simulink model "MCU_CmdTransV3"  (R2022b)
settings: Solver=FixedStepDiscrete  StartTime=0.0  StopTime=10.0  FixedStep=0.001  RelTol=1e-3
undefined symbols (not defined in the file or in its folder): ANALOG, cAgeingMode, cCurrentLoopMode, cNoneMode, cParaRecogMode, cSingleBoardMode, cSpeedLoopMode, cTorqueLoopMode, cVvvfOpenMode, FAULT, ParamCfg_CommandSource_u16, ParamCfg_MaxSpeed_u16, ParamCfg_MaxTorque_u16, ParamCfg_Spdouttype_u16, ParamCfg_Vc1Enable_u16, POWER_ON, STANDBY, TESTBED, VEHICLE
libraries: simulink x8
(part 1 of 2)
settings Model: DataDictionary=MCU_CmdTransV2_objects.sldd  Creator=ZYH  LastModifiedBy=ZYH
settings OptimizationCC: DefaultParameterBehavior=Inlined  EnhancedBackFolding=on  PassReuseOutputArgsAs=Individual arguments  OptimizeBlockOrder=speed  DifferentSizesBufferReuse=on  OptimizationCustomize=off  EfficientTunableParamExpr=on
settings DebuggingCC: ParameterTunabilityLossMsg=error
settings SFSimCC: MATLABDynamicMemAlloc=off
settings RTWCC: Description=Embedded Coder  SystemTargetFile=ert.tlc  GenCodeOnly=on  TemplateMakefile=ert_default_tmf
settings CodeAppCC: ForceParamTrailComments=on  IgnoreCustomStorageClasses=off  OperatorAnnotations=on  SimulinkDataObjDesc=on  SFDataObjDesc=on  InsertBlockDesc=on
settings ERTTargetCC: TargetLangStandard=C99 (ISO)  GenerateSampleERTMain=on  InlinedParameterPlacement=NonHierarchical  ERTCustomFileTemplate=example_file_process.tlc

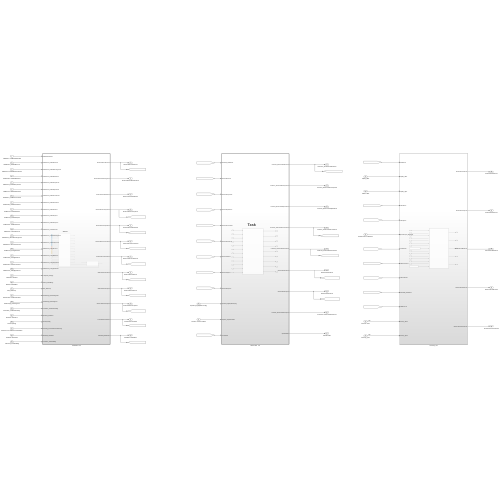
[thumbnail: Simulink's stored preview of the top-level diagram]
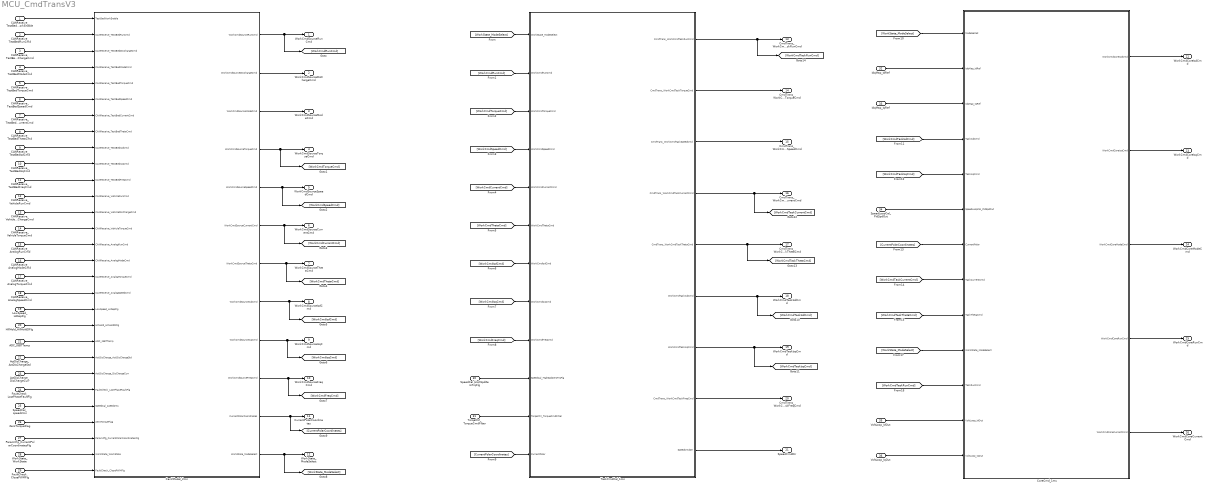
== system MCU_CmdTransV3 ==
  CANReceive_TestBedWorkEnable : Inport
  CANReceive_TestBedRunCmd : Inport  Port=2
  CANReceive_TestBedDisChargeCmd : Inport  Port=3
  CANReceive_TestBedModeCmd : Inport  Port=4
  CANReceive_TestBedTorqueCmd : Inport  Port=5
  CANReceive_TestBedSpeedCmd : Inport  Port=6
  CANReceive_TestBedCurrentCmd : Inport  Port=7
  CANReceive_TestBedThetaCmd : Inport  Port=8
  CANReceive_TestBedIsdCmd : Inport  Port=9
  CANReceive_TestBedIsqCmd : Inport  Port=10
  CANReceive_TestBedFreqCmd : Inport  Port=11
  CANReceive_VehicleRunCmd : Inport  Port=12
  CANReceive_VehicleDisChargeCmd : Inport  Port=13
  CANReceive_VehicleTorqueCmd : Inport  Port=14
  CANReceive_AnalogRunCmd : Inport  Port=15
  CANReceive_AnalogModeCmd : Inport  Port=16
  CANReceive_AnalogTorqueCmd : Inport  Port=17
  CANReceive_AnalogSpeedCmd : Inport  Port=18
  LowSpeed_LsDepFlg : Inport  Port=19
  HillHold_HillHoldDFlg : Inport  Port=20
  ADC_IGBTTemp : Inport  Port=21
  ActDisCharge_ActDisChargeStd : Inport  Port=22
  ActDisCharge_DisChargeCurr : Inport  Port=23
  FaultCheck_LostPhaseFaultFlg : Inport  Port=24
  SpeedCal_speed2ms : Inport  Port=25
  ZeroTorqueFlag : Inport  Port=26
  ParamCfg_CurrentPolarCoordinatesFlg : Inport  Port=27
  WorkState_WorkState : Inport  Port=28
  FaultCheck_ClosePWMFlg : Inport  Port=29
  SpeedCal_HighSpdZeroTrqFlg : Inport  Port=30
  TorqeCtrl_TorqueCmdFilter : Inport  Port=31
  IdqMap_IdRef : Inport  Port=32
  IdqMap_IqRef : Inport  Port=33
  SpeedLoopCal_PidSpdOut : Inport  Port=34
  VoltLoop_IdOut : Inport  Port=35  OutDataTypeStr=single
  VoltLoop_IqOut : Inport  Port=36  OutDataTypeStr=single
  Can2Model_2ms : Subsystem  TreatAsAtomicUnit=on
  CoreCmd_1ms : Subsystem
  TaskCmdCal_1ms : Subsystem  TreatAsAtomicUnit=on
  WorkCmdSourceRunCmd : Outport
  WorkCmdSourceDisChargeCmd : Outport  Port=2
  WorkCmdSourceModeCmd : Outport  Port=3
  WorkCmdSourceTorqueCmd : Outport  Port=4
  WorkCmdSourceSpeedCmd : Outport  Port=5
  WorkCmdSourceCurrentCmd : Outport  Port=6
  WorkCmdSourceThetaCmd : Outport  Port=7
  WorkCmdSourceIsdCmd : Outport  Port=8
  WorkCmdSourceIsqCmd : Outport  Port=9
  WorkCmdSourceFreqCmd : Outport  Port=10
  CurrentPolarCoordinates : Outport  Port=11
  WorkState_ModeSelect : Outport  Port=12
  CmdTrans_WorkCmdTaskRunCmd : Outport  Port=13
  CmdTrans_WorkCmdTaskTorqueCmd : Outport  Port=14
  CmdTrans_WorkCmdTaskSpeedCmd : Outport  Port=15
  CmdTrans_WorkCmdTaskCurrentCmd : Outport  Port=16
  CmdTrans_WorkCmdTaskThetaCmd : Outport  Port=17
  WorkCmdTaskIsdCmd : Outport  Port=18
  WorkCmdTaskIsqCmd : Outport  Port=19
  CmdTrans_WorkCmdTaskFreqCmd : Outport  Port=20
  SpeedCmdDir : Outport  Port=21
  WorkCmdCoreIsdCmd : Outport  Port=22
  WorkCmdCoreIsqCmd : Outport  Port=23
  WorkCmdCoreModeCmd : Outport  Port=24
  WorkCmdCoreRunCmd : Outport  Port=25
  WorkCmdCoreCurrentCmd : Outport  Port=26
  wires:
  CANReceive_TestBedModeCmd/1 -> Can2Model_2ms/4(CANReceive_TestBedModeCmd)
  CANReceive_TestBedTorqueCmd/1 -> Can2Model_2ms/5(CANReceive_TestBedTorqueCmd)
  CANReceive_TestBedDisChargeCmd/1 -> Can2Model_2ms/3(CANReceive_TestBedDisChargeCmd)
  CANReceive_TestBedWorkEnable/1 -> Can2Model_2ms/1(TestBedWorkEnable)
  CANReceive_TestBedRunCmd/1 -> Can2Model_2ms/2(CANReceive_TestBedRunCmd)
  CANReceive_TestBedIsdCmd/1 -> Can2Model_2ms/9(CANReceive_TestBedIsdCmd)
  CANReceive_TestBedIsqCmd/1 -> Can2Model_2ms/10(CANReceive_TestBedIsqCmd)
  CANReceive_TestBedThetaCmd/1 -> Can2Model_2ms/8(CANReceive_TestBedThetaCmd)
  CANReceive_TestBedFreqCmd/1 -> Can2Model_2ms/11(CANReceive_TestBedFreqCmd)
  CANReceive_VehicleRunCmd/1 -> Can2Model_2ms/12(CANReceive_VehicleRunCmd)
  CANReceive_VehicleDisChargeCmd/1 -> Can2Model_2ms/13(CANReceive_VehicleDisChargeCmd)
  CANReceive_TestBedCurrentCmd/1 -> Can2Model_2ms/7(CANReceive_TestBedCurrentCmd)
  CANReceive_TestBedSpeedCmd/1 -> Can2Model_2ms/6(CANReceive_TestBedSpeedCmd)
  CANReceive_AnalogTorqueCmd/1 -> Can2Model_2ms/17(CANReceive_AnalogTorqueCmd)
  CANReceive_AnalogSpeedCmd/1 -> Can2Model_2ms/18(CANReceive_AnalogSpeedCmd)
  CANReceive_AnalogModeCmd/1 -> Can2Model_2ms/16(CANReceive_AnalogModeCmd)
  LowSpeed_LsDepFlg/1 -> Can2Model_2ms/19(LowSpeed_LsDepFlg)
  CANReceive_AnalogRunCmd/1 -> Can2Model_2ms/15(CANReceive_AnalogRunCmd)
  CANReceive_VehicleTorqueCmd/1 -> Can2Model_2ms/14(CANReceive_VehicleTorqueCmd)
  ActDisCharge_ActDisChargeStd/1 -> Can2Model_2ms/22(ActDisCharge_ActDisChargeStd)
  ActDisCharge_DisChargeCurr/1 -> Can2Model_2ms/23(ActDisCharge_DisChargeCurr)
  FaultCheck_LostPhaseFaultFlg/1 -> Can2Model_2ms/24(FaultCheck_LostPhaseFaultFlg)
  Can2Model_2ms/1(WorkCmdSourceRunCmd) -> [WorkCmdRunCmd], WorkCmdSourceRunCmd/1
  Can2Model_2ms/2(WorkCmdSourceDisChargeCmd) -> WorkCmdSourceDisChargeCmd/1
  Can2Model_2ms/3(WorkCmdSourceModeCmd) -> WorkCmdSourceModeCmd/1
  Can2Model_2ms/4(WorkCmdSourceTorqueCmd) -> [WorkCmdTorqueCmd], WorkCmdSourceTorqueCmd/1
  Can2Model_2ms/5(WorkCmdSourceSpeedCmd) -> WorkCmdSourceSpeedCmd/1, [WorkCmdSpeedCmd]
  Can2Model_2ms/6(WorkCmdSourceCurrentCmd) -> WorkCmdSourceCurrentCmd/1, [WorkCmdCurrentCmd]
  Can2Model_2ms/7(WorkCmdSourceThetaCmd) -> WorkCmdSourceThetaCmd/1, [WorkCmdThetaCmd]
  Can2Model_2ms/8(WorkCmdSourceIsdCmd) -> WorkCmdSourceIsdCmd/1, [WorkCmdIsdCmd]
  Can2Model_2ms/9(WorkCmdSourceIsqCmd) -> [WorkCmdIsqCmd], WorkCmdSourceIsqCmd/1
  Can2Model_2ms/11(CurrentPolarCoordinates) -> [CurrentPolarCoordinates], CurrentPolarCoordinates/1
  Can2Model_2ms/10(WorkCmdSourceFreqCmd) -> [WorkCmdFreqCmd], WorkCmdSourceFreqCmd/1
  ParamCfg_CurrentPolarCoordinatesFlg/1 -> Can2Model_2ms/27(ParamCfg_CurrentPolarCoordinatesFlg)
  ZeroTorqueFlag/1 -> Can2Model_2ms/26(ZeroTorqueFlag)
  SpeedCal_speed2ms/1 -> Can2Model_2ms/25(SpeedCal_speed2ms)
  WorkState_WorkState/1 -> Can2Model_2ms/28(WorkState_WorkState)
  FaultCheck_ClosePWMFlg/1 -> Can2Model_2ms/29(FaultCheck_ClosePWMFlg)
  Can2Model_2ms/12(WorkState_ModeSelect) -> [WorkState_ModeSelect], WorkState_ModeSelect/1
  [WorkState_ModeSelect] -> TaskCmdCal_1ms/1(WorkState_ModeSelect)
  [WorkCmdRunCmd] -> TaskCmdCal_1ms/2(WorkCmdRunCmd)
  [WorkCmdTorqueCmd] -> TaskCmdCal_1ms/3(WorkCmdTorqueCmd)
  [WorkCmdSpeedCmd] -> TaskCmdCal_1ms/4(WorkCmdSpeedCmd)
  [WorkCmdCurrentCmd] -> TaskCmdCal_1ms/5(WorkCmdCurrentCmd)
  [WorkCmdThetaCmd] -> TaskCmdCal_1ms/6(WorkCmdThetaCmd)
  [WorkCmdIsdCmd] -> TaskCmdCal_1ms/7(WorkCmdIsdCmd)
  [WorkCmdIsqCmd] -> TaskCmdCal_1ms/8(WorkCmdIsqCmd)
  [WorkCmdFreqCmd] -> TaskCmdCal_1ms/9(WorkCmdFreqCmd)
  SpeedCal_HighSpdZeroTrqFlg/1 -> TaskCmdCal_1ms/10(SpeedCal_HighSpdZeroTrqFlg)
  TorqeCtrl_TorqueCmdFilter/1 -> TaskCmdCal_1ms/11(TorqeCtrl_TorqueCmdFilter)
  [CurrentPolarCoordinates] -> TaskCmdCal_1ms/12(CurrentPolar)
  HillHold_HillHoldDFlg/1 -> Can2Model_2ms/20(HillHold_HillHoldDFlg)
  ADC_IGBTTemp/1 -> Can2Model_2ms/21(ADC_IGBTTemp)
  TaskCmdCal_1ms/9(SpeedCmdDir) -> SpeedCmdDir/1
  TaskCmdCal_1ms/3(CmdTrans_WorkCmdTaskSpeedCmd) -> CmdTrans_WorkCmdTaskSpeedCmd/1
  TaskCmdCal_1ms/8(CmdTrans_WorkCmdTaskFreqCmd) -> CmdTrans_WorkCmdTaskFreqCmd/1
  TaskCmdCal_1ms/6(WorkCmdTaskIsdCmd) -> [WorkCmdTaskIsdCmd], WorkCmdTaskIsdCmd/1
  TaskCmdCal_1ms/5(CmdTrans_WorkCmdTaskThetaCmd) -> [WorkCmdTaskThetaCmd], CmdTrans_WorkCmdTaskThetaCmd/1
  TaskCmdCal_1ms/7(WorkCmdTaskIsqCmd) -> [WorkCmdTaskIsqCmd], WorkCmdTaskIsqCmd/1
  TaskCmdCal_1ms/2(CmdTrans_WorkCmdTaskTorqueCmd) -> CmdTrans_WorkCmdTaskTorqueCmd/1
  [WorkState_ModeSelect] -> CoreCmd_1ms/1(ModeSelcet)
  IdqMap_IdRef/1 -> CoreCmd_1ms/2(IdqMap_IdRef)
  IdqMap_IqRef/1 -> CoreCmd_1ms/3(IdqMap_IqRef)
  [WorkCmdTaskIsdCmd] -> CoreCmd_1ms/4(TaskIsdCmd)
  [WorkCmdTaskIsqCmd] -> CoreCmd_1ms/5(TaskIsqCmd)
  SpeedLoopCal_PidSpdOut/1 -> CoreCmd_1ms/6(SpeedLoopCal_PidSpdOut)
  VoltLoop_IdOut/1 -> CoreCmd_1ms/12(VoltLoop_IdOut)
  VoltLoop_IqOut/1 -> CoreCmd_1ms/13(VoltLoop_IqOut)
  [CurrentPolarCoordinates] -> CoreCmd_1ms/7(CurrentPolar)
  TaskCmdCal_1ms/4(CmdTrans_WorkCmdTaskCurrentCmd) -> [WorkCmdTaskCurrentCmd], CmdTrans_WorkCmdTaskCurrentCmd/1
  [WorkCmdTaskCurrentCmd] -> CoreCmd_1ms/8(TaskCurrentCmd)
  [WorkCmdTaskThetaCmd] -> CoreCmd_1ms/9(TaskThetaCmd)
  TaskCmdCal_1ms/1(CmdTrans_WorkCmdTaskRunCmd) -> [WorkCmdTaskRunCmd], CmdTrans_WorkCmdTaskRunCmd/1
  [WorkCmdTaskRunCmd] -> CoreCmd_1ms/11(TaskRunCmd)
  [WorkState_ModeSelect] -> CoreCmd_1ms/10(WorkState_ModeSelect)
  CoreCmd_1ms/1(WorkCmdCoreIsdCmd) -> WorkCmdCoreIsdCmd/1
  CoreCmd_1ms/2(WorkCmdCoreIsqCmd) -> WorkCmdCoreIsqCmd/1
  CoreCmd_1ms/3(WorkCmdCoreModeCmd) -> WorkCmdCoreModeCmd/1
  CoreCmd_1ms/4(WorkCmdCoreRunCmd) -> WorkCmdCoreRunCmd/1
  CoreCmd_1ms/5(WorkCmdCoreCurrentCmd) -> WorkCmdCoreCurrentCmd/1

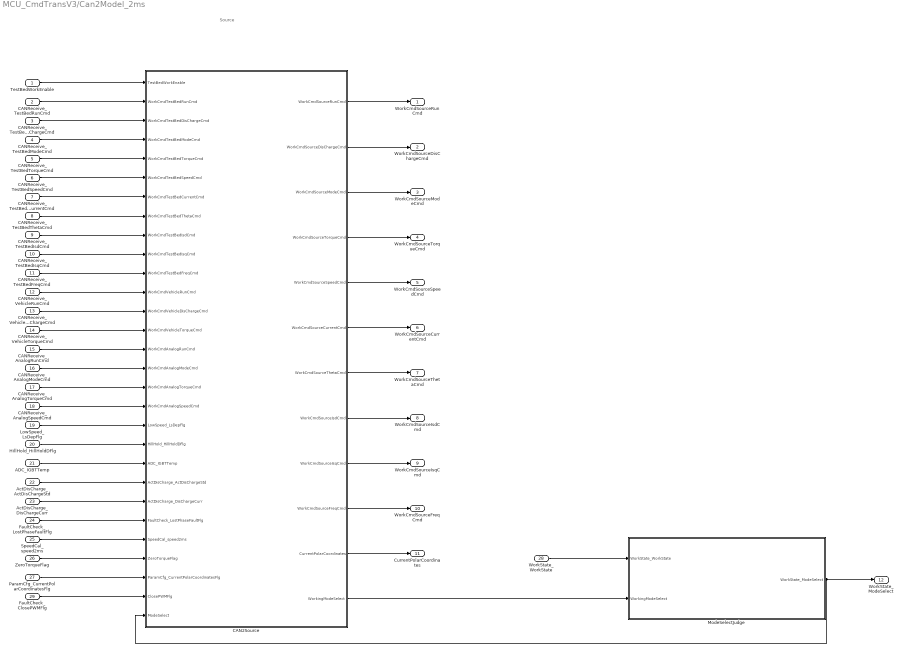
== system MCU_CmdTransV3/Can2Model_2ms ==
  note: Source
  TestBedWorkEnable : Inport
  CANReceive_TestBedRunCmd : Inport  Port=2
  CANReceive_TestBedDisChargeCmd : Inport  Port=3
  CANReceive_TestBedModeCmd : Inport  Port=4
  CANReceive_TestBedTorqueCmd : Inport  Port=5
  CANReceive_TestBedSpeedCmd : Inport  Port=6
  CANReceive_TestBedCurrentCmd : Inport  Port=7
  CANReceive_TestBedThetaCmd : Inport  Port=8
  CANReceive_TestBedIsdCmd : Inport  Port=9
  CANReceive_TestBedIsqCmd : Inport  Port=10
  CANReceive_TestBedFreqCmd : Inport  Port=11
  CANReceive_VehicleRunCmd : Inport  Port=12
  CANReceive_VehicleDisChargeCmd : Inport  Port=13
  CANReceive_VehicleTorqueCmd : Inport  Port=14
  CANReceive_AnalogRunCmd : Inport  Port=15
  CANReceive_AnalogModeCmd : Inport  Port=16
  CANReceive_AnalogTorqueCmd : Inport  Port=17
  CANReceive_AnalogSpeedCmd : Inport  Port=18
  LowSpeed_LsDepFlg : Inport  Port=19
  HillHold_HillHoldDFlg : Inport  Port=20
  ADC_IGBTTemp : Inport  Port=21
  ActDisCharge_ActDisChargeStd : Inport  Port=22
  ActDisCharge_DisChargeCurr : Inport  Port=23
  FaultCheck_LostPhaseFaultFlg : Inport  Port=24
  SpeedCal_speed2ms : Inport  Port=25
  ZeroTorqueFlag : Inport  Port=26
  ParamCfg_CurrentPolarCoordinatesFlg : Inport  Port=27
  WorkState_WorkState : Inport  Port=28
  FaultCheck_ClosePWMFlg : Inport  Port=29
  CAN2Source : Subsystem  TreatAsAtomicUnit=on
      settings: RTWSystemCode=Nonreusable function
  ModeSelectJudge : Subsystem  TreatAsAtomicUnit=on
      settings: RTWSystemCode=Nonreusable function
  WorkCmdSourceRunCmd : Outport
  WorkCmdSourceDisChargeCmd : Outport  Port=2
  WorkCmdSourceModeCmd : Outport  Port=3
  WorkCmdSourceTorqueCmd : Outport  Port=4
  WorkCmdSourceSpeedCmd : Outport  Port=5
  WorkCmdSourceCurrentCmd : Outport  Port=6
  WorkCmdSourceThetaCmd : Outport  Port=7
  WorkCmdSourceIsdCmd : Outport  Port=8
  WorkCmdSourceIsqCmd : Outport  Port=9
  WorkCmdSourceFreqCmd : Outport  Port=10
  CurrentPolarCoordinates : Outport  Port=11
  WorkState_ModeSelect : Outport  Port=12
  wires:
  CANReceive_TestBedTorqueCmd/1 -> CAN2Source/5(WorkCmdTestBedTorqueCmd)
  CANReceive_TestBedIsdCmd/1 -> CAN2Source/9(WorkCmdTestBedIsdCmd)
  CANReceive_TestBedIsqCmd/1 -> CAN2Source/10(WorkCmdTestBedIsqCmd)
  LowSpeed_LsDepFlg/1 -> CAN2Source/19(LowSpeed_LsDepFlg)
  FaultCheck_LostPhaseFaultFlg/1 -> CAN2Source/24(FaultCheck_LostPhaseFaultFlg)
  CANReceive_AnalogModeCmd/1 -> CAN2Source/16(WorkCmdAnalogModeCmd)
  CANReceive_AnalogTorqueCmd/1 -> CAN2Source/17(WorkCmdAnalogTorqueCmd)
  CAN2Source/5(WorkCmdSourceSpeedCmd) -> WorkCmdSourceSpeedCmd/1
  CANReceive_VehicleTorqueCmd/1 -> CAN2Source/14(WorkCmdVehicleTorqueCmd)
  CANReceive_VehicleRunCmd/1 -> CAN2Source/12(WorkCmdVehicleRunCmd)
  ActDisCharge_DisChargeCurr/1 -> CAN2Source/23(ActDisCharge_DisChargeCurr)
  CANReceive_TestBedCurrentCmd/1 -> CAN2Source/7(WorkCmdTestBedCurrentCmd)
  CANReceive_TestBedFreqCmd/1 -> CAN2Source/11(WorkCmdTestBedFreqCmd)
  CAN2Source/10(WorkCmdSourceFreqCmd) -> WorkCmdSourceFreqCmd/1
  CAN2Source/3(WorkCmdSourceModeCmd) -> WorkCmdSourceModeCmd/1
  CAN2Source/7(WorkCmdSourceThetaCmd) -> WorkCmdSourceThetaCmd/1
  CANReceive_AnalogSpeedCmd/1 -> CAN2Source/18(WorkCmdAnalogSpeedCmd)
  CANReceive_TestBedRunCmd/1 -> CAN2Source/2(WorkCmdTestBedRunCmd)
  CAN2Source/4(WorkCmdSourceTorqueCmd) -> WorkCmdSourceTorqueCmd/1
  CANReceive_VehicleDisChargeCmd/1 -> CAN2Source/13(WorkCmdVehicleDisChargeCmd)
  TestBedWorkEnable/1 -> CAN2Source/1(TestBedWorkEnable)
  CANReceive_TestBedDisChargeCmd/1 -> CAN2Source/3(WorkCmdTestBedDisChargeCmd)
  CAN2Source/11(CurrentPolarCoordinates) -> CurrentPolarCoordinates/1
  CANReceive_AnalogRunCmd/1 -> CAN2Source/15(WorkCmdAnalogRunCmd)
  CANReceive_TestBedThetaCmd/1 -> CAN2Source/8(WorkCmdTestBedThetaCmd)
  CAN2Source/9(WorkCmdSourceIsqCmd) -> WorkCmdSourceIsqCmd/1
  ActDisCharge_ActDisChargeStd/1 -> CAN2Source/22(ActDisCharge_ActDisChargeStd)
  CAN2Source/1(WorkCmdSourceRunCmd) -> WorkCmdSourceRunCmd/1
  CAN2Source/6(WorkCmdSourceCurrentCmd) -> WorkCmdSourceCurrentCmd/1
  CANReceive_TestBedModeCmd/1 -> CAN2Source/4(WorkCmdTestBedModeCmd)
  CAN2Source/2(WorkCmdSourceDisChargeCmd) -> WorkCmdSourceDisChargeCmd/1
  CAN2Source/8(WorkCmdSourceIsdCmd) -> WorkCmdSourceIsdCmd/1
  CANReceive_TestBedSpeedCmd/1 -> CAN2Source/6(WorkCmdTestBedSpeedCmd)
  ModeSelectJudge/1(WorkState_ModeSelect) -> WorkState_ModeSelect/1, CAN2Source/29(ModeSelect)
  SpeedCal_speed2ms/1 -> CAN2Source/25(SpeedCal_speed2ms)
  ParamCfg_CurrentPolarCoordinatesFlg/1 -> CAN2Source/27(ParamCfg_CurrentPolarCoordinatesFlg)
  ZeroTorqueFlag/1 -> CAN2Source/26(ZeroTorqueFlag)
  CAN2Source/12(WorkingModeSelect) -> ModeSelectJudge/2(WorkingModeSelect)
  WorkState_WorkState/1 -> ModeSelectJudge/1(WorkState_WorkState)
  FaultCheck_ClosePWMFlg/1 -> CAN2Source/28(ClosePWMFlg)
  ADC_IGBTTemp/1 -> CAN2Source/21(ADC_IGBTTemp)
  HillHold_HillHoldDFlg/1 -> CAN2Source/20(HillHold_HillHoldDFlg)

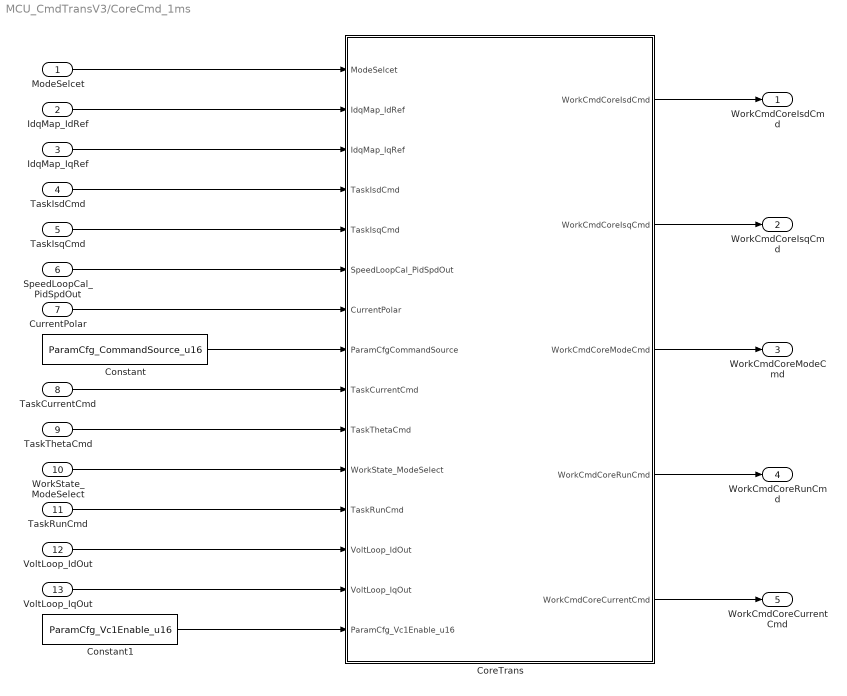
== system MCU_CmdTransV3/CoreCmd_1ms ==
  ModeSelcet : Inport
  IdqMap_IdRef : Inport  Port=2
  IdqMap_IqRef : Inport  Port=3
  TaskIsdCmd : Inport  Port=4
  TaskIsqCmd : Inport  Port=5
  SpeedLoopCal_PidSpdOut : Inport  Port=6
  CurrentPolar : Inport  Port=7
  TaskCurrentCmd : Inport  Port=8
  TaskThetaCmd : Inport  Port=9
  WorkState_ModeSelect : Inport  Port=10
  TaskRunCmd : Inport  Port=11
  VoltLoop_IdOut : Inport  Port=12
  VoltLoop_IqOut : Inport  Port=13
  Constant : Constant  Value=ParamCfg_CommandSource_u16
  Constant1 : Constant  Value=ParamCfg_Vc1Enable_u16
  CoreTrans : Subsystem
  WorkCmdCoreIsdCmd : Outport
  WorkCmdCoreIsqCmd : Outport  Port=2
  WorkCmdCoreModeCmd : Outport  Port=3
  WorkCmdCoreRunCmd : Outport  Port=4
  WorkCmdCoreCurrentCmd : Outport  Port=5
  wires:
  ModeSelcet/1 -> CoreTrans/1(ModeSelcet)
  TaskIsdCmd/1 -> CoreTrans/4(TaskIsdCmd)
  IdqMap_IqRef/1 -> CoreTrans/3(IdqMap_IqRef)
  TaskIsqCmd/1 -> CoreTrans/5(TaskIsqCmd)
  SpeedLoopCal_PidSpdOut/1 -> CoreTrans/6(SpeedLoopCal_PidSpdOut)
  CurrentPolar/1 -> CoreTrans/7(CurrentPolar)
  IdqMap_IdRef/1 -> CoreTrans/2(IdqMap_IdRef)
  TaskCurrentCmd/1 -> CoreTrans/9(TaskCurrentCmd)
  TaskThetaCmd/1 -> CoreTrans/10(TaskThetaCmd)
  WorkState_ModeSelect/1 -> CoreTrans/11(WorkState_ModeSelect)
  TaskRunCmd/1 -> CoreTrans/12(TaskRunCmd)
  VoltLoop_IdOut/1 -> CoreTrans/13(VoltLoop_IdOut)
  Constant/1 -> CoreTrans/8(ParamCfgCommandSource)
  VoltLoop_IqOut/1 -> CoreTrans/14(VoltLoop_IqOut)
  Constant1/1 -> CoreTrans/15(ParamCfg_Vc1Enable_u16)
  CoreTrans/1(WorkCmdCoreIsdCmd) -> WorkCmdCoreIsdCmd/1
  CoreTrans/5(WorkCmdCoreCurrentCmd) -> WorkCmdCoreCurrentCmd/1
  CoreTrans/4(WorkCmdCoreRunCmd) -> WorkCmdCoreRunCmd/1
  CoreTrans/3(WorkCmdCoreModeCmd) -> WorkCmdCoreModeCmd/1
  CoreTrans/2(WorkCmdCoreIsqCmd) -> WorkCmdCoreIsqCmd/1

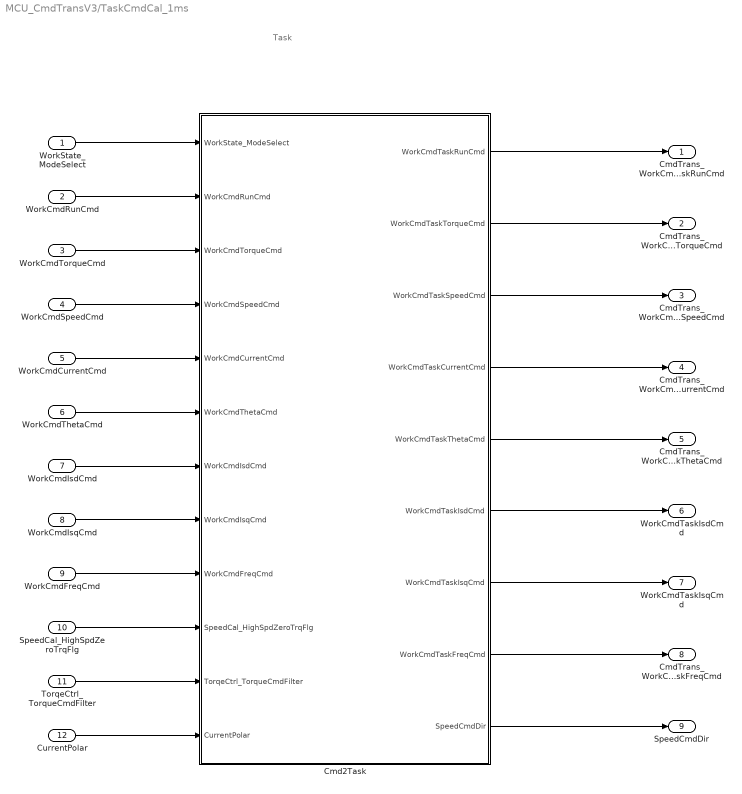
== system MCU_CmdTransV3/TaskCmdCal_1ms ==
  note: Task
  WorkState_ModeSelect : Inport
  WorkCmdRunCmd : Inport  Port=2
  WorkCmdTorqueCmd : Inport  Port=3
  WorkCmdSpeedCmd : Inport  Port=4
  WorkCmdCurrentCmd : Inport  Port=5
  WorkCmdThetaCmd : Inport  Port=6
  WorkCmdIsdCmd : Inport  Port=7
  WorkCmdIsqCmd : Inport  Port=8
  WorkCmdFreqCmd : Inport  Port=9
  SpeedCal_HighSpdZeroTrqFlg : Inport  Port=10
  TorqeCtrl_TorqueCmdFilter : Inport  Port=11
  CurrentPolar : Inport  Port=12
  Cmd2Task : Subsystem
  CmdTrans_WorkCmdTaskRunCmd : Outport
  CmdTrans_WorkCmdTaskTorqueCmd : Outport  Port=2
  CmdTrans_WorkCmdTaskSpeedCmd : Outport  Port=3
  CmdTrans_WorkCmdTaskCurrentCmd : Outport  Port=4
  CmdTrans_WorkCmdTaskThetaCmd : Outport  Port=5
  WorkCmdTaskIsdCmd : Outport  Port=6
  WorkCmdTaskIsqCmd : Outport  Port=7
  CmdTrans_WorkCmdTaskFreqCmd : Outport  Port=8
  SpeedCmdDir : Outport  Port=9
  wires:
  WorkState_ModeSelect/1 -> Cmd2Task/1(WorkState_ModeSelect)
  WorkCmdRunCmd/1 -> Cmd2Task/2(WorkCmdRunCmd)
  WorkCmdTorqueCmd/1 -> Cmd2Task/3(WorkCmdTorqueCmd)
  WorkCmdSpeedCmd/1 -> Cmd2Task/4(WorkCmdSpeedCmd)
  WorkCmdCurrentCmd/1 -> Cmd2Task/5(WorkCmdCurrentCmd)
  WorkCmdThetaCmd/1 -> Cmd2Task/6(WorkCmdThetaCmd)
  WorkCmdIsdCmd/1 -> Cmd2Task/7(WorkCmdIsdCmd)
  WorkCmdIsqCmd/1 -> Cmd2Task/8(WorkCmdIsqCmd)
  WorkCmdFreqCmd/1 -> Cmd2Task/9(WorkCmdFreqCmd)
  SpeedCal_HighSpdZeroTrqFlg/1 -> Cmd2Task/10(SpeedCal_HighSpdZeroTrqFlg)
  TorqeCtrl_TorqueCmdFilter/1 -> Cmd2Task/11(TorqeCtrl_TorqueCmdFilter)
  CurrentPolar/1 -> Cmd2Task/12(CurrentPolar)
  Cmd2Task/1(WorkCmdTaskRunCmd) -> CmdTrans_WorkCmdTaskRunCmd/1
  Cmd2Task/2(WorkCmdTaskTorqueCmd) -> CmdTrans_WorkCmdTaskTorqueCmd/1
  Cmd2Task/3(WorkCmdTaskSpeedCmd) -> CmdTrans_WorkCmdTaskSpeedCmd/1
  Cmd2Task/4(WorkCmdTaskCurrentCmd) -> CmdTrans_WorkCmdTaskCurrentCmd/1
  Cmd2Task/5(WorkCmdTaskThetaCmd) -> CmdTrans_WorkCmdTaskThetaCmd/1
  Cmd2Task/8(WorkCmdTaskFreqCmd) -> CmdTrans_WorkCmdTaskFreqCmd/1
  Cmd2Task/9(SpeedCmdDir) -> SpeedCmdDir/1
  Cmd2Task/6(WorkCmdTaskIsdCmd) -> WorkCmdTaskIsdCmd/1
  Cmd2Task/7(WorkCmdTaskIsqCmd) -> WorkCmdTaskIsqCmd/1

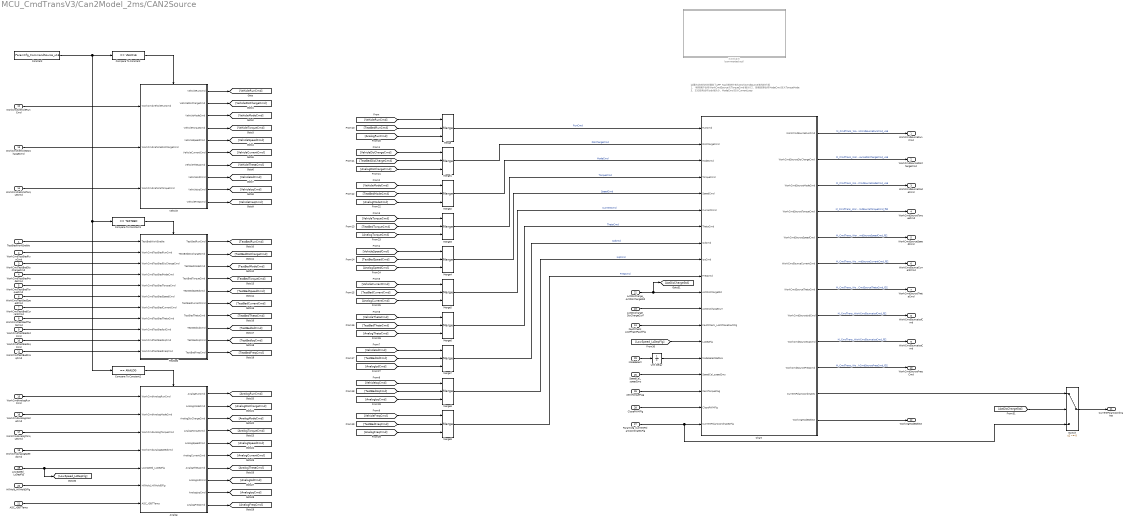
== system MCU_CmdTransV3/Can2Model_2ms/CAN2Source ==
  note: 这里的状态机时处理除了APP_Task模块外有对WorkCmdSource修改的代码
      | 1、·堵转保护会将WorkCmdSource的TorqueCmd赋为0
      | 2、缺相故障会将ModeCmd改为TorqueMode
      | 3、主动放电会将Isdq赋为0，ModeCmd改为CurrentLoop
  TestBedWorkEnable : Inport
  WorkCmdTestBedRunCmd : Inport  Port=2
  WorkCmdTestBedDisChargeCmd : Inport  Port=3
  WorkCmdTestBedModeCmd : Inport  Port=4
  WorkCmdTestBedTorqueCmd : Inport  Port=5
  WorkCmdTestBedSpeedCmd : Inport  Port=6
  WorkCmdTestBedCurrentCmd : Inport  Port=7
  WorkCmdTestBedThetaCmd : Inport  Port=8
  WorkCmdTestBedIsdCmd : Inport  Port=9
  WorkCmdTestBedIsqCmd : Inport  Port=10
  WorkCmdTestBedFreqCmd : Inport  Port=11
  WorkCmdVehicleRunCmd : Inport  Port=12
  WorkCmdVehicleDisChargeCmd : Inport  Port=13
  WorkCmdVehicleTorqueCmd : Inport  Port=14
  WorkCmdAnalogRunCmd : Inport  Port=15
  WorkCmdAnalogModeCmd : Inport  Port=16
  WorkCmdAnalogTorqueCmd : Inport  Port=17
  WorkCmdAnalogSpeedCmd : Inport  Port=18
  LowSpeed_LsDepFlg : Inport  Port=19
  HillHold_HillHoldDFlg : Inport  Port=20
  ADC_IGBTTemp : Inport  Port=21
  ActDisCharge_ActDisChargeStd : Inport  Port=22
  ActDisCharge_DisChargeCurr : Inport  Port=23
  FaultCheck_LostPhaseFaultFlg : Inport  Port=24
  SpeedCal_speed2ms : Inport  Port=25
  ZeroTorqueFlag : Inport  Port=26
  ParamCfg_CurrentPolarCoordinatesFlg : Inport  Port=27
  ClosePWMFlg : Inport  Port=28
  ModeSelect : Inport  Port=29
  Analog : Subsystem  TreatAsAtomicUnit=on
  Chart : Stateflow chart  TreatAsAtomicUnit=on
      settings: PortSchema="{\"entries\":[{\"content\":{\"sides\":[{\"content\":{\"connectorIds\":[\"In1\",\"In2\",\"In3\",\"In4\",\"In5\",\"In6\",\"In7\",\"In8\",\"In9\",\"In10\",\"In11\",\"In12\",\"In13\",\"In14\",\"In15\",\"In16\",\"In17\",\"In19\",\"In18\"]},\"type\":\"ConnectorPlacement.EquallySpacedRectSide\",\"uuid\":\"7fc2b22f-11a9-4923-9e5c-cd0c66c11027\"},{\"content\":{\"connectorIds\":[\"Out1\",\"Out2\",\"Out3\",\"Out4\",\"Out5\",\"Out6\",\"Out7\",\"Out8\",\"Out9\",\"Out10\",\"Out11\",\"Out12\"],\"side\":\"RIGHT\"},\"type\":\"ConnectorPlacement.EquallySpacedRectSide\",\"uuid\":\"0fded8e1-5396-4642-832c-285206fbc267\"},{\"content\":{\"connectorIds\":[],\"side\":\"TOP\"},\"type\":\"ConnectorPlacement.EquallySpacedRectSide\",\"uuid\":\"51014235-5064-478a-94f6-3a61d1f546c3\"}]},\"type\":\"ConnectorPlacement.EquallySpacedConnector\",\"uuid\":\"ff4f0e04-a0fb-4bac-acc5-90c954e511bb\"}],\"packageUris\":[\"http://schema.mathworks.com/mf0/Connector/R2020b\"],\"version\":\"1.0\"}"
  Compare To Constant : simulink/Logic and Bit Operations/Compare To Constant  relop===  const=VEHICLE  OutDataTypeStr=boolean
  Compare To Constant1 : simulink/Logic and Bit Operations/Compare To Constant  relop===  const=TESTBED  OutDataTypeStr=boolean
  Compare To Constant2 : simulink/Logic and Bit Operations/Compare To Constant  relop===  const=ANALOG  OutDataTypeStr=boolean
  Constant : Constant  Value=ParamCfg_CommandSource_u16
  Merge{,1..9} (10 alike) : Merge  Inputs=3
  Switch : Switch  Criteria=u2 ~= 0  SaturateOnIntegerOverflow=off  InputSameDT=off
  Testbed : Subsystem  TreatAsAtomicUnit=on
  Unit Delay : UnitDelay  SampleTime=-1  HasFrameUpgradeWarning=on
  Vehicle : Subsystem
  状态机备份 : Subsystem  Commented=on
  WorkCmdSourceRunCmd : Outport
  WorkCmdSourceDisChargeCmd : Outport  Port=2
  WorkCmdSourceModeCmd : Outport  Port=3
  WorkCmdSourceTorqueCmd : Outport  Port=4
  WorkCmdSourceSpeedCmd : Outport  Port=5
  WorkCmdSourceCurrentCmd : Outport  Port=6
  WorkCmdSourceThetaCmd : Outport  Port=7
  WorkCmdSourceIsdCmd : Outport  Port=8
  WorkCmdSourceIsqCmd : Outport  Port=9
  WorkCmdSourceFreqCmd : Outport  Port=10
  CurrentPolarCoordinates : Outport  Port=11
  WorkingModeSelect : Outport  Port=12
  wires:
  Constant/1 -> Compare To Constant2/1, Compare To Constant1/1, Compare To Constant/1
  Compare To Constant/1 -> Vehicle/Enable
  WorkCmdVehicleRunCmd/1 -> Vehicle/1(WorkCmdVehicleRunCmd)
  WorkCmdVehicleDisChargeCmd/1 -> Vehicle/2(WorkCmdVehicleDisChargeCmd)
  WorkCmdVehicleTorqueCmd/1 -> Vehicle/3(WorkCmdVehicleTorqueCmd)
  Compare To Constant1/1 -> Testbed/Enable
  WorkCmdTestBedModeCmd/1 -> Testbed/4(WorkCmdTestBedModeCmd)
  WorkCmdTestBedTorqueCmd/1 -> Testbed/5(WorkCmdTestBedTorqueCmd)
  WorkCmdTestBedDisChargeCmd/1 -> Testbed/3(WorkCmdTestBedDisChargeCmd)
  WorkCmdTestBedSpeedCmd/1 -> Testbed/6(WorkCmdTestBedSpeedCmd)
  WorkCmdTestBedRunCmd/1 -> Testbed/2(WorkCmdTestBedRunCmd)
  WorkCmdTestBedCurrentCmd/1 -> Testbed/7(WorkCmdTestBedCurrentCmd)
  WorkCmdTestBedThetaCmd/1 -> Testbed/8(WorkCmdTestBedThetaCmd)
  WorkCmdTestBedIsdCmd/1 -> Testbed/9(WorkCmdTestBedIsdCmd)
  WorkCmdTestBedIsqCmd/1 -> Testbed/10(WorkCmdTestBedIsqCmd)
  WorkCmdTestBedFreqCmd/1 -> Testbed/11(WorkCmdTestBedFreqCmd)
  Compare To Constant2/1 -> Analog/Enable
  WorkCmdAnalogRunCmd/1 -> Analog/1(WorkCmdAnalogRunCmd)
  WorkCmdAnalogModeCmd/1 -> Analog/2(WorkCmdAnalogModeCmd)
  WorkCmdAnalogTorqueCmd/1 -> Analog/3(WorkCmdAnalogTorqueCmd)
  WorkCmdAnalogSpeedCmd/1 -> Analog/4(WorkCmdAnalogSpeedCmd)
  TestBedWorkEnable/1 -> Testbed/1(TestBedWorkEnable)
  Vehicle/1(VehicleRunCmd) -> [VehicleRunCmd]
  Vehicle/2(VehicleDisChargeCmd) -> [VehicleDisChargeCmd]
  Vehicle/3(VehicleModeCmd) -> [VehicleModeCmd]
  Vehicle/4(VehicleTorqueCmd) -> [VehicleTorqueCmd]
  Vehicle/5(VehicleSpeedCmd) -> [VehicleSpeedCmd]
  Vehicle/6(VehicleCurrentCmd) -> [VehicleCurrentCmd]
  Vehicle/7(VehicleThetaCmd) -> [VehicleThetaCmd]
  Vehicle/8(VehicleIsdCmd) -> [VehicleIsdCmd]
  Vehicle/9(VehicleIsqCmd) -> [VehicleIsqCmd]
  Vehicle/10(VehicleFreqCmd) -> [VehicleFreqCmd]
  Testbed/2(TestBedDisChargeCmd) -> [TestBedDisChargeCmd]
  Testbed/3(TestBedModeCmd) -> [TestBedModeCmd]
  Testbed/4(TestBedTorqueCmd) -> [TestBedTorqueCmd]
  Testbed/5(TestBedSpeedCmd) -> [TestBedSpeedCmd]
  Testbed/6(TestBedCurrentCmd) -> [TestBedCurrentCmd]
  Testbed/7(TestBedThetaCmd) -> [TestBedThetaCmd]
  Testbed/8(TestBedIsdCmd) -> [TestBedIsdCmd]
  Testbed/9(TestBedIsqCmd) -> [TestBedIsqCmd]
  Testbed/10(TestBedFreqCmd) -> [TestBedFreqCmd]
  Testbed/1(TestBedRunCmd) -> [TestBedRunCmd]
  Analog/2(AnalogModeCmd) -> [AnalogDisChargeCmd]
  Analog/3(AnalogDisChargeCmd) -> [AnalogModeCmd]
  Analog/4(AnalogTorqueCmd) -> [AnalogTorqueCmd]
  Analog/5(AnalogSpeedCmd) -> [AnalogSpeedCmd]
  Analog/6(AnalogCurrentCmd) -> [AnalogCurrentCmd]
  Analog/7(AnalogThetaCmd) -> [AnalogThetaCmd]
  Analog/8(AnalogIsdCmd) -> [AnalogIsdCmd]
  Analog/9(AnalogIsqCmd) -> [AnalogIsqCmd]
  Analog/10(AnalogFreqCmd) -> [AnalogFreqCmd]
  Analog/1(AnalogRunCmd) -> [AnalogRunCmd]
  [VehicleRunCmd] -> Merge/1
  [VehicleDisChargeCmd] -> Merge1/1
  [VehicleModeCmd] -> Merge2/1
  [VehicleTorqueCmd] -> Merge3/1
  [VehicleSpeedCmd] -> Merge4/1
  [VehicleFreqCmd] -> Merge9/1
  [VehicleCurrentCmd] -> Merge5/1
  [VehicleThetaCmd] -> Merge6/1
  [VehicleIsdCmd] -> Merge7/1
  [VehicleIsqCmd] -> Merge8/1
  [TestBedRunCmd] -> Merge/2
  [TestBedDisChargeCmd] -> Merge1/2
  [TestBedModeCmd] -> Merge2/2
  [TestBedTorqueCmd] -> Merge3/2
  [TestBedSpeedCmd] -> Merge4/2
  [TestBedCurrentCmd] -> Merge5/2
  [TestBedThetaCmd] -> Merge6/2
  [TestBedIsdCmd] -> Merge7/2
  [TestBedIsqCmd] -> Merge8/2
  [TestBedFreqCmd] -> Merge9/2
  [AnalogFreqCmd] -> Merge9/3
  [AnalogRunCmd] -> Merge/3
  [AnalogDisChargeCmd] -> Merge1/3
  [AnalogModeCmd] -> Merge2/3
  [AnalogTorqueCmd] -> Merge3/3
  [AnalogSpeedCmd] -> Merge4/3
  [AnalogCurrentCmd] -> Merge5/3
  [AnalogThetaCmd] -> Merge6/3
  [AnalogIsdCmd] -> Merge7/3
  [AnalogIsqCmd] -> Merge8/3
  Merge/1 -> Chart/1(RunCmd)  "RunCmd"
  Merge1/1 -> Chart/2(DisChargeCmd)  "DisChargeCmd"
  Merge2/1 -> Chart/3(ModeCmd)  "ModeCmd"
  Merge3/1 -> Chart/4(TorqueCmd)  "TorqueCmd"
  Merge4/1 -> Chart/5(SpeedCmd)  "SpeedCmd"
  Merge5/1 -> Chart/6(CurrentCmd)  "CurrentCmd"
  Merge6/1 -> Chart/7(ThetaCmd)  "ThetaCmd"
  Merge7/1 -> Chart/8(IsdCmd)  "IsdCmd"
  Merge8/1 -> Chart/9(IsqCmd)  "IsqCmd"
  Merge9/1 -> Chart/10(FreqCmd)  "FreqCmd"
  LowSpeed_LsDepFlg/1 -> [LowSpeed_LsDepFlg], Analog/5(LowSpeed_LsDepFlg)
  Chart/1(WorkCmdSourceRunCmd) -> WorkCmdSourceRunCmd/1  "M_CmdTrans_WorkCmdSourceRunCmd_u16"
  Chart/2(WorkCmdSourceDisChargeCmd) -> WorkCmdSourceDisChargeCmd/1  "M_CmdTrans_WorkCmdSourceDisChargeCmd_u16"
  Chart/3(WorkCmdSourceModeCmd) -> WorkCmdSourceModeCmd/1  "M_CmdTrans_WorkCmdSourceModeCmd_u16"
  Chart/4(WorkCmdSourceTorqueCmd) -> WorkCmdSourceTorqueCmd/1  "M_CmdTrans_WorkCmdSourceTorqueCmd_f32"
  Chart/5(WorkCmdSourceSpeedCmd) -> WorkCmdSourceSpeedCmd/1  "M_CmdTrans_WorkCmdSourceSpeedCmd_f32"
  Chart/6(WorkCmdSourceCurrentCmd) -> WorkCmdSourceCurrentCmd/1  "M_CmdTrans_WorkCmdSourceCurrentCmd_f32"
  Chart/7(WorkCmdSourceThetaCmd) -> WorkCmdSourceThetaCmd/1  "M_CmdTrans_WorkCmdSourceThetaCmd_f32"
  Chart/8(WorkCmdSourceIsdCmd) -> WorkCmdSourceIsdCmd/1  "M_CmdTrans_WorkCmdSourceIsdCmd_f32"
  Chart/9(WorkCmdSourceIsqCmd) -> WorkCmdSourceIsqCmd/1  "M_CmdTrans_WorkCmdSourceIsqCmd_f32"
  Chart/10(WorkCmdSourceFreqCmd) -> WorkCmdSourceFreqCmd/1  "M_CmdTrans_WorkCmdSourceFreqCmd_f32"
  ActDisCharge_ActDisChargeStd/1 -> [ActDisChargeStd], Chart/11(ActDisChargeStd)
  ActDisCharge_DisChargeCurr/1 -> Chart/12(ActDisChargeCurr)
  FaultCheck_LostPhaseFaultFlg/1 -> Chart/13(FaultCheck_LostPhaseFaultFlg)
  [LowSpeed_LsDepFlg] -> Chart/14(LsDepFlg)
  Chart/11(CurrentPolarCoordinates) -> Switch/1
  Chart/12(WorkingModeSelect) -> WorkingModeSelect/1
  ModeSelect/1 -> Unit Delay/1
  SpeedCal_speed2ms/1 -> Chart/16(SpeedCal_speed2ms)
  ZeroTorqueFlag/1 -> Chart/17(ZeroTorqueFlag)
  ParamCfg_CurrentPolarCoordinatesFlg/1 -> Switch/3, Chart/18(CurrentPolarCoordinatesFlg)
  Unit Delay/1 -> Chart/15(ModeSelectBefore)
  ClosePWMFlg/1 -> Chart/19(ClosePWMFlg)
  [ActDisChargeStd] -> Switch/2
  Switch/1 -> CurrentPolarCoordinates/1
  HillHold_HillHoldDFlg/1 -> Analog/6(HillHold_HillHoldDFlg)
  ADC_IGBTTemp/1 -> Analog/7(ADC_IGBTTemp)

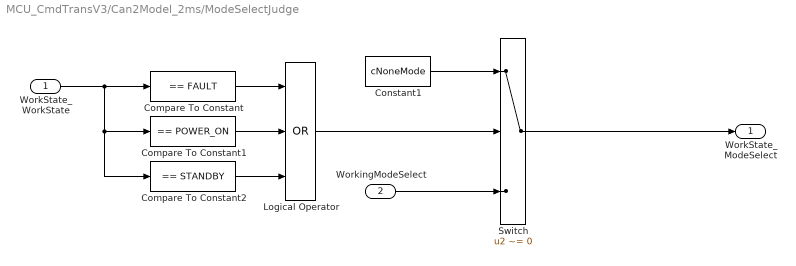
== system MCU_CmdTransV3/Can2Model_2ms/ModeSelectJudge ==
  WorkState_WorkState : Inport
  WorkingModeSelect : Inport  Port=2
  Compare To Constant : simulink/Logic and Bit Operations/Compare To Constant  relop===  const=FAULT  OutDataTypeStr=boolean
  Compare To Constant1 : simulink/Logic and Bit Operations/Compare To Constant  relop===  const=POWER_ON  OutDataTypeStr=boolean
  Compare To Constant2 : simulink/Logic and Bit Operations/Compare To Constant  relop===  const=STANDBY  OutDataTypeStr=boolean
  Constant1 : Constant  Value=cNoneMode  VectorParams1D=off  OutDataTypeStr=uint16
  Logical Operator : Logic  Operator=OR  Inputs=3  AllPortsSameDT=off  OutDataTypeStr=boolean
  Switch : Switch  Criteria=u2 ~= 0  SaturateOnIntegerOverflow=off  InputSameDT=off
  WorkState_ModeSelect : Outport
  wires:
  Constant1/1 -> Switch/1
  Compare To Constant/1 -> Logical Operator/1
  Logical Operator/1 -> Switch/2
  WorkState_WorkState/1 -> Compare To Constant2/1, Compare To Constant1/1, Compare To Constant/1
  Compare To Constant2/1 -> Logical Operator/3
  Compare To Constant1/1 -> Logical Operator/2
  WorkingModeSelect/1 -> Switch/3
  Switch/1 -> WorkState_ModeSelect/1

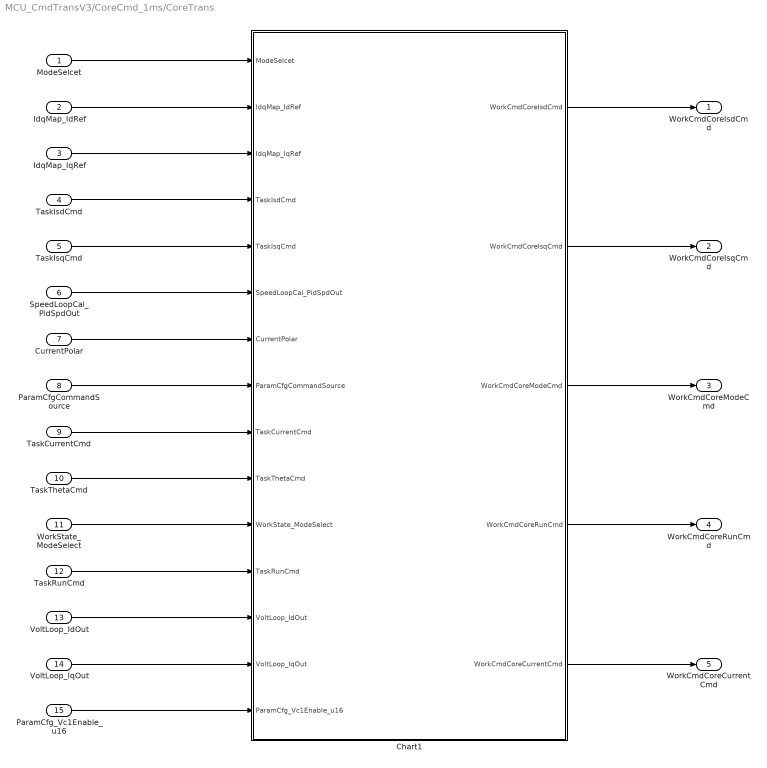
== system MCU_CmdTransV3/CoreCmd_1ms/CoreTrans ==
  ModeSelcet : Inport
  IdqMap_IdRef : Inport  Port=2
  IdqMap_IqRef : Inport  Port=3
  TaskIsdCmd : Inport  Port=4
  TaskIsqCmd : Inport  Port=5
  SpeedLoopCal_PidSpdOut : Inport  Port=6
  CurrentPolar : Inport  Port=7
  ParamCfgCommandSource : Inport  Port=8
  TaskCurrentCmd : Inport  Port=9
  TaskThetaCmd : Inport  Port=10
  WorkState_ModeSelect : Inport  Port=11
  TaskRunCmd : Inport  Port=12
  VoltLoop_IdOut : Inport  Port=13
  VoltLoop_IqOut : Inport  Port=14
  ParamCfg_Vc1Enable_u16 : Inport  Port=15
  Chart1 : Stateflow chart  TreatAsAtomicUnit=on
  WorkCmdCoreIsdCmd : Outport
  WorkCmdCoreIsqCmd : Outport  Port=2
  WorkCmdCoreModeCmd : Outport  Port=3
  WorkCmdCoreRunCmd : Outport  Port=4
  WorkCmdCoreCurrentCmd : Outport  Port=5
  wires:
  ModeSelcet/1 -> Chart1/1(ModeSelcet)
  IdqMap_IdRef/1 -> Chart1/2(IdqMap_IdRef)
  IdqMap_IqRef/1 -> Chart1/3(IdqMap_IqRef)
  TaskIsqCmd/1 -> Chart1/5(TaskIsqCmd)
  SpeedLoopCal_PidSpdOut/1 -> Chart1/6(SpeedLoopCal_PidSpdOut)
  TaskIsdCmd/1 -> Chart1/4(TaskIsdCmd)
  CurrentPolar/1 -> Chart1/7(CurrentPolar)
  ParamCfgCommandSource/1 -> Chart1/8(ParamCfgCommandSource)
  TaskThetaCmd/1 -> Chart1/10(TaskThetaCmd)
  WorkState_ModeSelect/1 -> Chart1/11(WorkState_ModeSelect)
  TaskCurrentCmd/1 -> Chart1/9(TaskCurrentCmd)
  TaskRunCmd/1 -> Chart1/12(TaskRunCmd)
  VoltLoop_IdOut/1 -> Chart1/13(VoltLoop_IdOut)
  VoltLoop_IqOut/1 -> Chart1/14(VoltLoop_IqOut)
  ParamCfg_Vc1Enable_u16/1 -> Chart1/15(ParamCfg_Vc1Enable_u16)
  Chart1/5(WorkCmdCoreCurrentCmd) -> WorkCmdCoreCurrentCmd/1
  Chart1/1(WorkCmdCoreIsdCmd) -> WorkCmdCoreIsdCmd/1
  Chart1/4(WorkCmdCoreRunCmd) -> WorkCmdCoreRunCmd/1
  Chart1/2(WorkCmdCoreIsqCmd) -> WorkCmdCoreIsqCmd/1
  Chart1/3(WorkCmdCoreModeCmd) -> WorkCmdCoreModeCmd/1

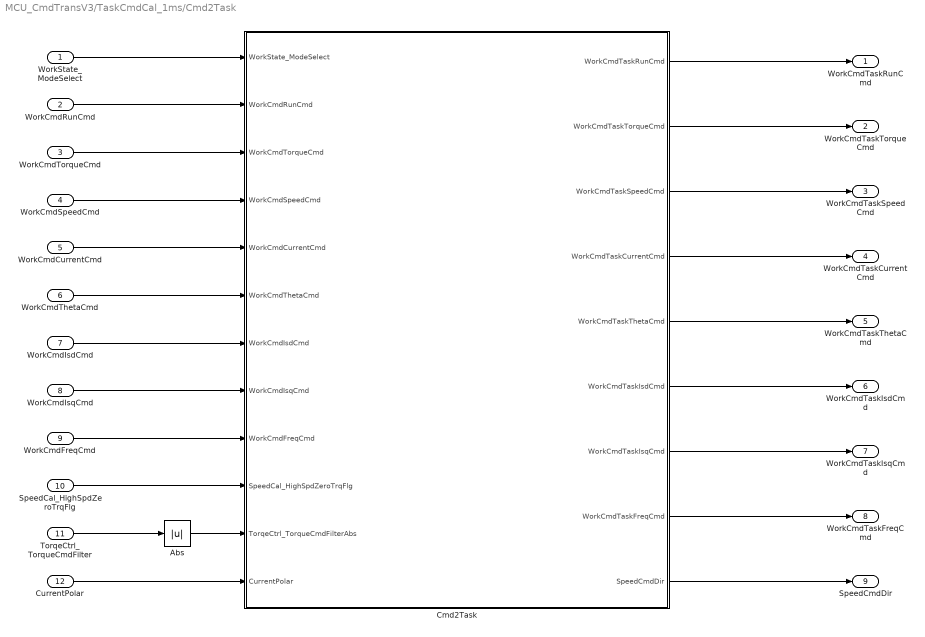
== system MCU_CmdTransV3/TaskCmdCal_1ms/Cmd2Task ==
  WorkState_ModeSelect : Inport
  WorkCmdRunCmd : Inport  Port=2
  WorkCmdTorqueCmd : Inport  Port=3
  WorkCmdSpeedCmd : Inport  Port=4
  WorkCmdCurrentCmd : Inport  Port=5
  WorkCmdThetaCmd : Inport  Port=6
  WorkCmdIsdCmd : Inport  Port=7
  WorkCmdIsqCmd : Inport  Port=8
  WorkCmdFreqCmd : Inport  Port=9
  SpeedCal_HighSpdZeroTrqFlg : Inport  Port=10
  TorqeCtrl_TorqueCmdFilter : Inport  Port=11
  CurrentPolar : Inport  Port=12
  Abs : Abs  SaturateOnIntegerOverflow=off
  Cmd2Task : Stateflow chart  TreatAsAtomicUnit=on
      settings: PortSchema="{\"entries\":[{\"content\":{\"sides\":[{\"content\":{\"connectorIds\":[\"In2\",\"In3\",\"In4\",\"In5\",\"In6\",\"In7\",\"In1\",\"In8\",\"In9\",\"In10\",\"In11\",\"In12\"]},\"type\":\"ConnectorPlacement.EquallySpacedRectSide\",\"uuid\":\"3aeab0a9-977f-4d7e-9da7-61fabe5cb386\"},{\"content\":{\"connectorIds\":[\"Out1\",\"Out2\",\"Out3\",\"Out4\",\"Out5\",\"Out6\",\"Out7\",\"Out8\",\"Out9\"],\"side\":\"RIGHT\"},\"type\":\"ConnectorPlacement.EquallySpacedRectSide\",\"uuid\":\"52d65e32-3a7d-4d72-b988-d1b9ef3f3299\"},{\"content\":{\"connectorIds\":[],\"side\":\"TOP\"},\"type\":\"ConnectorPlacement.EquallySpacedRectSide\",\"uuid\":\"7eee4f92-79ee-4dfc-b51c-d644466ec602\"},{\"content\":{\"connectorIds\":[],\"side\":\"BOTTOM\"},\"type\":\"ConnectorPlacement.EquallySpacedRectSide\",\"uuid\":\"a847cf42-6c44-46d8-9270-33361270c7f2\"}]},\"type\":\"ConnectorPlacement.EquallySpacedConnector\",\"uuid\":\"d7c8bde0-45fa-4435-a641-175901423035\"}],\"packageUris\":[\"http://schema.mathworks.com/mf0/Connector/R2020b\"],\"version\":\"1.0\"}"
  WorkCmdTaskRunCmd : Outport
  WorkCmdTaskTorqueCmd : Outport  Port=2
  WorkCmdTaskSpeedCmd : Outport  Port=3
  WorkCmdTaskCurrentCmd : Outport  Port=4
  WorkCmdTaskThetaCmd : Outport  Port=5
  WorkCmdTaskIsdCmd : Outport  Port=6
  WorkCmdTaskIsqCmd : Outport  Port=7
  WorkCmdTaskFreqCmd : Outport  Port=8
  SpeedCmdDir : Outport  Port=9
  wires:
  Cmd2Task/8(WorkCmdTaskFreqCmd) -> WorkCmdTaskFreqCmd/1
  CurrentPolar/1 -> Cmd2Task/12(CurrentPolar)
  Abs/1 -> Cmd2Task/11(TorqeCtrl_TorqueCmdFilterAbs)
  Cmd2Task/2(WorkCmdTaskTorqueCmd) -> WorkCmdTaskTorqueCmd/1
  WorkCmdRunCmd/1 -> Cmd2Task/3(WorkCmdRunCmd)
  Cmd2Task/6(WorkCmdTaskIsdCmd) -> WorkCmdTaskIsdCmd/1
  SpeedCal_HighSpdZeroTrqFlg/1 -> Cmd2Task/10(SpeedCal_HighSpdZeroTrqFlg)
  WorkCmdIsqCmd/1 -> Cmd2Task/8(WorkCmdIsqCmd)
  Cmd2Task/4(WorkCmdTaskCurrentCmd) -> WorkCmdTaskCurrentCmd/1
  WorkCmdFreqCmd/1 -> Cmd2Task/9(WorkCmdFreqCmd)
  WorkCmdCurrentCmd/1 -> Cmd2Task/6(WorkCmdCurrentCmd)
  WorkCmdSpeedCmd/1 -> Cmd2Task/5(WorkCmdSpeedCmd)
  WorkCmdTorqueCmd/1 -> Cmd2Task/4(WorkCmdTorqueCmd)
  WorkCmdIsdCmd/1 -> Cmd2Task/1(WorkCmdIsdCmd)
  WorkState_ModeSelect/1 -> Cmd2Task/2(WorkState_ModeSelect)
  WorkCmdThetaCmd/1 -> Cmd2Task/7(WorkCmdThetaCmd)
  TorqeCtrl_TorqueCmdFilter/1 -> Abs/1
  Cmd2Task/5(WorkCmdTaskThetaCmd) -> WorkCmdTaskThetaCmd/1
  Cmd2Task/3(WorkCmdTaskSpeedCmd) -> WorkCmdTaskSpeedCmd/1
  Cmd2Task/9(SpeedCmdDir) -> SpeedCmdDir/1
  Cmd2Task/1(WorkCmdTaskRunCmd) -> WorkCmdTaskRunCmd/1
  Cmd2Task/7(WorkCmdTaskIsqCmd) -> WorkCmdTaskIsqCmd/1

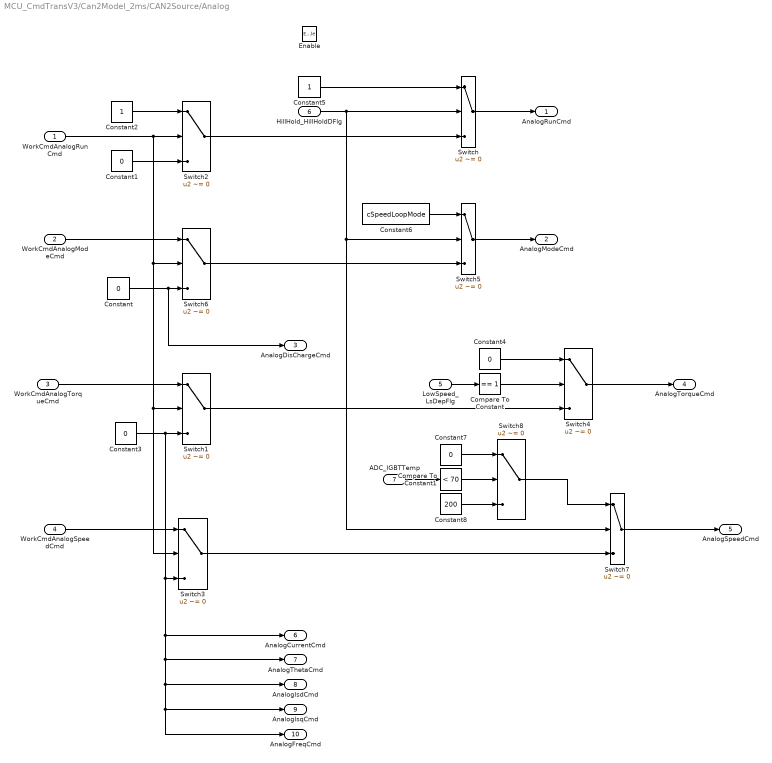
== system MCU_CmdTransV3/Can2Model_2ms/CAN2Source/Analog ==
  WorkCmdAnalogRunCmd : Inport
  WorkCmdAnalogModeCmd : Inport  Port=2
  WorkCmdAnalogTorqueCmd : Inport  Port=3
  WorkCmdAnalogSpeedCmd : Inport  Port=4
  LowSpeed_LsDepFlg : Inport  Port=5
  HillHold_HillHoldDFlg : Inport  Port=6
  ADC_IGBTTemp : Inport  Port=7
  Enable : EnablePort
  Compare To Constant : simulink/Logic and Bit Operations/Compare To Constant  relop===  const=1  OutDataTypeStr=boolean
  Compare To Constant1 : simulink/Logic and Bit Operations/Compare To Constant  relop=<  const=70  OutDataTypeStr=boolean
  Constant : Constant  Value=0  OutDataTypeStr=uint16
  Constant1 : Constant  Value=0  OutDataTypeStr=uint16
  Constant2 : Constant  OutDataTypeStr=uint16
  Constant3 : Constant  Value=0  OutDataTypeStr=single
  Constant4 : Constant  Value=0  OutDataTypeStr=single
  Constant5 : Constant  OutDataTypeStr=uint16
  Constant6 : Constant  Value=cSpeedLoopMode
  Constant7 : Constant  Value=0  OutDataTypeStr=single
  Constant8 : Constant  Value=200  OutDataTypeStr=single
  Switch{,1..8} (9 alike) : Switch  Criteria=u2 ~= 0  SaturateOnIntegerOverflow=off  InputSameDT=off
  AnalogRunCmd : Outport
  AnalogModeCmd : Outport  Port=2
  AnalogDisChargeCmd : Outport  Port=3
  AnalogTorqueCmd : Outport  Port=4
  AnalogSpeedCmd : Outport  Port=5
  AnalogCurrentCmd : Outport  Port=6
  AnalogThetaCmd : Outport  Port=7
  AnalogIsdCmd : Outport  Port=8
  AnalogIsqCmd : Outport  Port=9
  AnalogFreqCmd : Outport  Port=10
  wires:
  WorkCmdAnalogRunCmd/1 -> Switch2/2, Switch3/2, Switch1/2, Switch6/2
  WorkCmdAnalogModeCmd/1 -> Switch6/1
  Switch6/1 -> Switch5/3
  Constant/1 -> AnalogDisChargeCmd/1, Switch6/3
  Switch2/1 -> Switch/3
  Constant1/1 -> Switch2/3
  Constant2/1 -> Switch2/1
  WorkCmdAnalogTorqueCmd/1 -> Switch1/1
  Switch1/1 -> Switch4/3
  WorkCmdAnalogSpeedCmd/1 -> Switch3/1
  Switch3/1 -> Switch7/3
  Constant3/1 -> AnalogCurrentCmd/1, AnalogThetaCmd/1, AnalogIsdCmd/1, AnalogIsqCmd/1, AnalogFreqCmd/1, Switch3/3, Switch1/3
  LowSpeed_LsDepFlg/1 -> Compare To Constant/1
  Compare To Constant/1 -> Switch4/2
  Switch4/1 -> AnalogTorqueCmd/1
  Constant4/1 -> Switch4/1
  HillHold_HillHoldDFlg/1 -> Switch/2, Switch7/2, Switch5/2
  Switch/1 -> AnalogRunCmd/1
  Constant5/1 -> Switch/1
  Switch5/1 -> AnalogModeCmd/1
  Constant6/1 -> Switch5/1
  ADC_IGBTTemp/1 -> Compare To Constant1/1
  Compare To Constant1/1 -> Switch8/2
  Constant7/1 -> Switch8/1
  Constant8/1 -> Switch8/3
  Switch8/1 -> Switch7/1
  Switch7/1 -> AnalogSpeedCmd/1

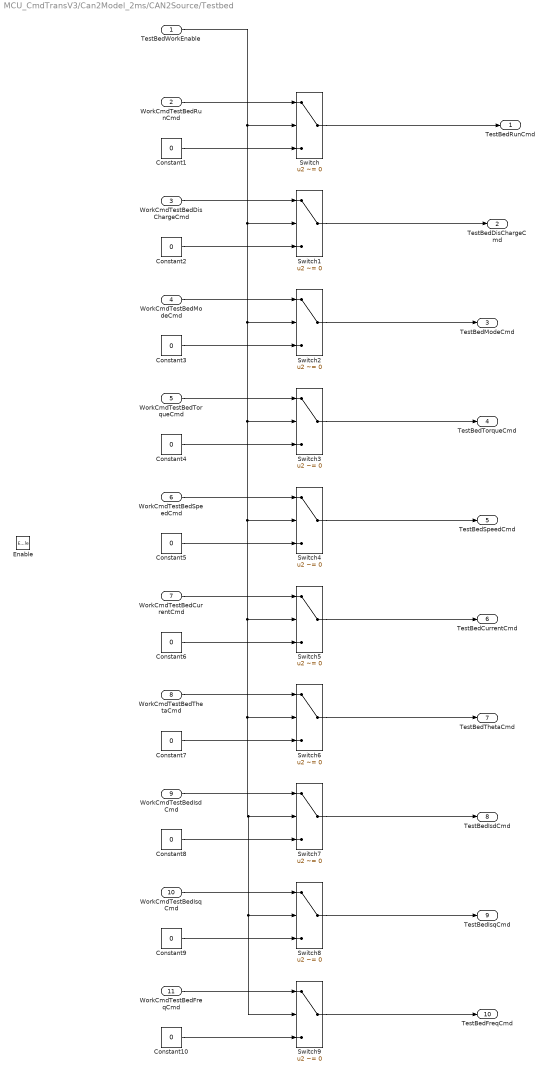
== system MCU_CmdTransV3/Can2Model_2ms/CAN2Source/Testbed ==
  TestBedWorkEnable : Inport
  WorkCmdTestBedRunCmd : Inport  Port=2
  WorkCmdTestBedDisChargeCmd : Inport  Port=3
  WorkCmdTestBedModeCmd : Inport  Port=4
  WorkCmdTestBedTorqueCmd : Inport  Port=5
  WorkCmdTestBedSpeedCmd : Inport  Port=6
  WorkCmdTestBedCurrentCmd : Inport  Port=7
  WorkCmdTestBedThetaCmd : Inport  Port=8
  WorkCmdTestBedIsdCmd : Inport  Port=9
  WorkCmdTestBedIsqCmd : Inport  Port=10
  WorkCmdTestBedFreqCmd : Inport  Port=11
  Enable : EnablePort
  Constant1 : Constant  Value=0  OutDataTypeStr=uint16
  Constant{4..10} (7 alike) : Constant  Value=0  OutDataTypeStr=single
  Constant2 : Constant  Value=0  OutDataTypeStr=uint16
  Constant3 : Constant  Value=0  OutDataTypeStr=uint16
  Switch{,1..9} (10 alike) : Switch  Criteria=u2 ~= 0  SaturateOnIntegerOverflow=off  InputSameDT=off
  TestBedRunCmd : Outport
  TestBedDisChargeCmd : Outport  Port=2
  TestBedModeCmd : Outport  Port=3
  TestBedTorqueCmd : Outport  Port=4
  TestBedSpeedCmd : Outport  Port=5
  TestBedCurrentCmd : Outport  Port=6
  TestBedThetaCmd : Outport  Port=7
  TestBedIsdCmd : Outport  Port=8
  TestBedIsqCmd : Outport  Port=9
  TestBedFreqCmd : Outport  Port=10
  wires:
  Constant1/1 -> Switch/3
  WorkCmdTestBedRunCmd/1 -> Switch/1
  WorkCmdTestBedDisChargeCmd/1 -> Switch1/1
  Constant2/1 -> Switch1/3
  WorkCmdTestBedModeCmd/1 -> Switch2/1
  Constant3/1 -> Switch2/3
  TestBedWorkEnable/1 -> Switch9/2, Switch8/2, Switch7/2, Switch6/2, Switch5/2, Switch4/2, Switch3/2, Switch2/2, Switch1/2, Switch/2
  WorkCmdTestBedTorqueCmd/1 -> Switch3/1
  Constant4/1 -> Switch3/3
  WorkCmdTestBedSpeedCmd/1 -> Switch4/1
  WorkCmdTestBedCurrentCmd/1 -> Switch5/1
  WorkCmdTestBedThetaCmd/1 -> Switch6/1
  WorkCmdTestBedIsdCmd/1 -> Switch7/1
  WorkCmdTestBedIsqCmd/1 -> Switch8/1
  WorkCmdTestBedFreqCmd/1 -> Switch9/1
  Constant5/1 -> Switch4/3
  Constant6/1 -> Switch5/3
  Constant7/1 -> Switch6/3
  Constant8/1 -> Switch7/3
  Constant9/1 -> Switch8/3
  Constant10/1 -> Switch9/3
  Switch/1 -> TestBedRunCmd/1
  Switch1/1 -> TestBedDisChargeCmd/1
  Switch2/1 -> TestBedModeCmd/1
  Switch3/1 -> TestBedTorqueCmd/1
  Switch4/1 -> TestBedSpeedCmd/1
  Switch5/1 -> TestBedCurrentCmd/1
  Switch6/1 -> TestBedThetaCmd/1
  Switch7/1 -> TestBedIsdCmd/1
  Switch8/1 -> TestBedIsqCmd/1
  Switch9/1 -> TestBedFreqCmd/1

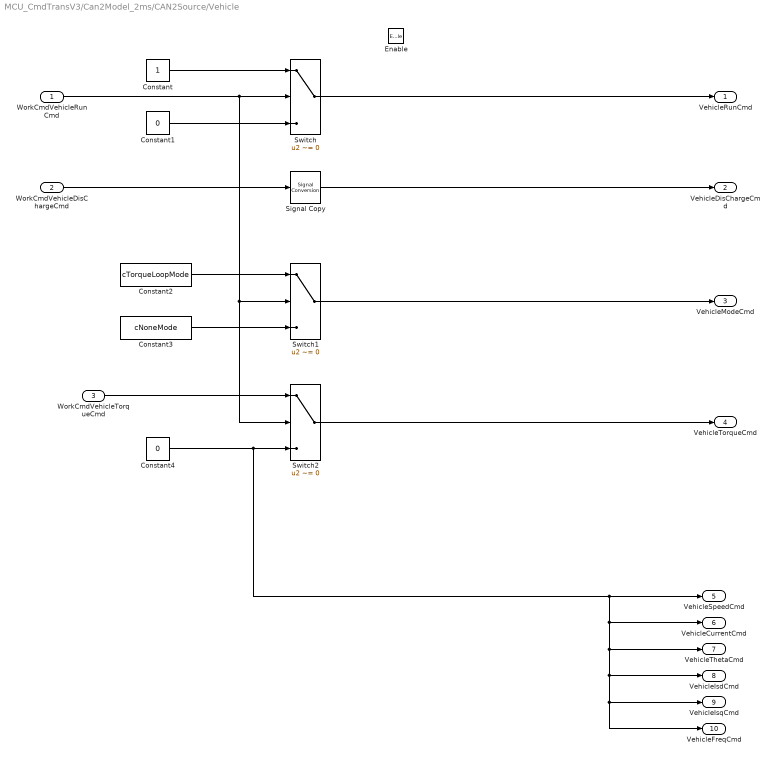
== system MCU_CmdTransV3/Can2Model_2ms/CAN2Source/Vehicle ==
  WorkCmdVehicleRunCmd : Inport
  WorkCmdVehicleDisChargeCmd : Inport  Port=2
  WorkCmdVehicleTorqueCmd : Inport  Port=3
  Enable : EnablePort
  Constant : Constant  OutDataTypeStr=uint16
  Constant1 : Constant  Value=0  OutDataTypeStr=uint16
  Constant2 : Constant  Value=cTorqueLoopMode
  Constant3 : Constant  Value=cNoneMode
  Constant4 : Constant  Value=0  OutDataTypeStr=single
  Signal Copy : SignalConversion  OverrideOpt=off
  Switch : Switch  Criteria=u2 ~= 0  SaturateOnIntegerOverflow=off  InputSameDT=off
  Switch1 : Switch  Criteria=u2 ~= 0  SaturateOnIntegerOverflow=off  InputSameDT=off
  Switch2 : Switch  Criteria=u2 ~= 0  SaturateOnIntegerOverflow=off  InputSameDT=off
  VehicleRunCmd : Outport
  VehicleDisChargeCmd : Outport  Port=2
  VehicleModeCmd : Outport  Port=3
  VehicleTorqueCmd : Outport  Port=4
  VehicleSpeedCmd : Outport  Port=5
  VehicleCurrentCmd : Outport  Port=6
  VehicleThetaCmd : Outport  Port=7
  VehicleIsdCmd : Outport  Port=8
  VehicleIsqCmd : Outport  Port=9
  VehicleFreqCmd : Outport  Port=10
  wires:
  WorkCmdVehicleRunCmd/1 -> Switch2/2, Switch1/2, Switch/2
  Constant/1 -> Switch/1
  Switch/1 -> VehicleRunCmd/1
  Constant1/1 -> Switch/3
  WorkCmdVehicleDisChargeCmd/1 -> Signal Copy/1
  Signal Copy/1 -> VehicleDisChargeCmd/1
  Constant2/1 -> Switch1/1
  Constant3/1 -> Switch1/3
  Switch1/1 -> VehicleModeCmd/1
  WorkCmdVehicleTorqueCmd/1 -> Switch2/1
  Constant4/1 -> VehicleThetaCmd/1, VehicleFreqCmd/1, VehicleIsqCmd/1, VehicleIsdCmd/1, VehicleCurrentCmd/1, VehicleSpeedCmd/1, Switch2/3
  Switch2/1 -> VehicleTorqueCmd/1

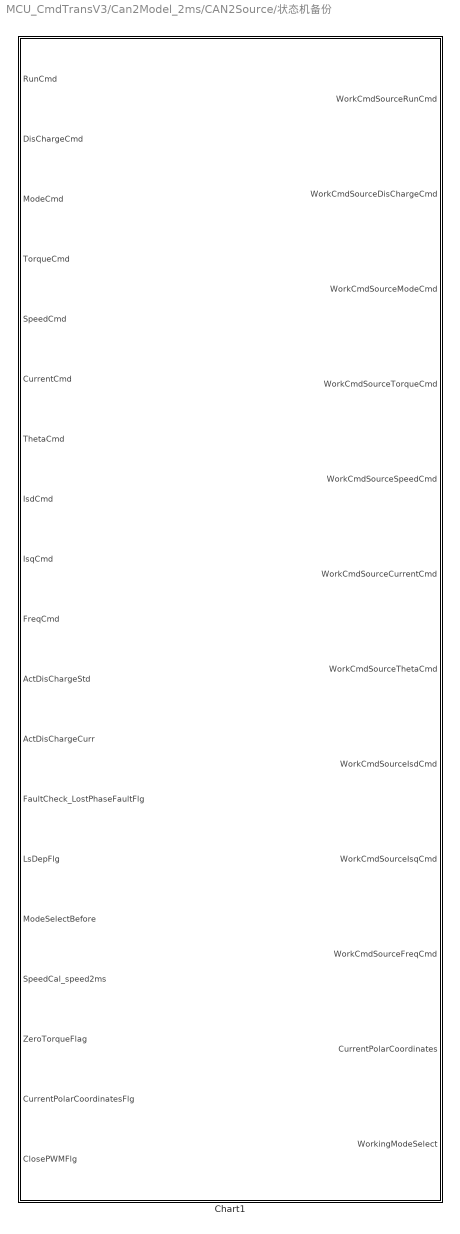
== system MCU_CmdTransV3/Can2Model_2ms/CAN2Source/状态机备份 ==
  Chart1 : Stateflow chart  TreatAsAtomicUnit=on

== stateflow chart MCU_CmdTransV3/CoreCmd_1ms/CoreTrans/Chart1 ==
  (default) -> (junction 8) : {
      | WorkCmdCoreIsdCmd = TaskIsdCmd;
      | WorkCmdCoreIsqCmd = TaskIsqCmd;
      | WorkCmdCoreModeCmd = WorkState_ModeSelect;
      | WorkCmdCoreRunCmd = TaskRunCmd;
      | }
  (junction 8) -> (junction 10) [order 1] : [(ModeSelcet == cTorqueLoopMode) || (ModeSelcet==cSpeedLoopMode && ParamCfg_Spdouttype_u16 == 0)]
      | {WorkCmdCoreIsdCmd = IdqMap_IdRef;
      | WorkCmdCoreIsqCmd  = IdqMap_IqRef}
  (junction 8) -> (junction 10) [order 2]
  (junction 10) -> (junction 18) [order 1] : [ModeSelcet == cSpeedLoopMode &&ParamCfg_Spdouttype_u16 ==1 ]
      | {
      | WorkCmdCoreIsdCmd = 0;
      | WorkCmdCoreIsqCmd = SpeedLoopCal_PidSpdOut;
      | }
  (junction 10) -> (junction 18) [order 2]
  (junction 18) -> (junction 22) [order 1] : [ModeSelcet == cCurrentLoopMode && CurrentPolar == 1 && ParamCfgCommandSource == TESTBED]
      | {
      | WorkCmdCoreIsdCmd = TaskCurrentCmd*sin(TaskThetaCmd)*(-1);
      | WorkCmdCoreIsqCmd = TaskCurrentCmd*cos(TaskThetaCmd);
      | }
  (junction 18) -> (junction 22) [order 2]
  (junction 22) -> (junction 36)
  (junction 36) -> (junction 35) [order 1] : [ParamCfg_Vc1Enable_u16 == 1 &&( ModeSelcet ==cTorqueLoopMode || (ModeSelcet ==cCurrentLoopMode && ParamCfgCommandSource == TESTBED))]
  (junction 36) -> (junction 37) [order 2]
  (junction 35) -> (junction 38) : {WorkCmdCoreIsdCmd=VoltLoop_IdOut
      | WorkCmdCoreIsqCmd = VoltLoop_IqOut}
  (junction 38) -> (junction 37)
  (junction 37) -> (junction 42) : {WorkCmdCoreCurrentCmd = sqrt(WorkCmdCoreIsdCmd * WorkCmdCoreIsdCmd + WorkCmdCoreIsqCmd * WorkCmdCoreIsqCmd)}
  (junction 42) -> (junction 55)
  data: ModeSelcet input; IdqMap_IdRef input single; IdqMap_IqRef input single; TaskIsdCmd input; TaskIsqCmd input; cSpeedLoopMode parameter; cTorqueLoopMode parameter; ParamCfg_Spdouttype_u16 parameter; SpeedLoopCal_PidSpdOut input single; cCurrentLoopMode parameter; CurrentPolar input; ParamCfgCommandSource input; TESTBED parameter; WorkCmdCoreIsdCmd output single =0; WorkCmdCoreIsqCmd output single =0; TaskCurrentCmd input; TaskThetaCmd input; WorkCmdCoreModeCmd output uint16 =cNoneMode; WorkState_ModeSelect input; TaskRunCmd input; VoltLoop_IdOut input; VoltLoop_IqOut input; WorkCmdCoreRunCmd output uint16 =0; ParamCfg_Vc1Enable_u16 input; WorkCmdCoreCurrentCmd output single =0
